simulink model "TRAS_PID_Pitch"  (R2016a)
settings: Solver=ode5  SolverMode=SingleTasking  StartTime=0.0  StopTime=90  FixedStep=0.01  RelTol=1e-3  AbsTol=1e-6
settings Model: SimulationMode=external  ExtModeTrigDuration=12000  ExtModeTrigLevel=0.400000  Creator=jims  LastModifiedBy=inteco
settings DataIOCC: ExternalInput=[]  InitialState=[]  MaxDataPoints=5000  SaveFormat=Array  SignalLoggingSaveFormat=ModelDataLogs  SaveOutput=off  SaveTime=off  SignalLoggingName=sigsOut
settings OptimizationCC: BooleanDataType=off  ExpressionDepthLimit=2147483647  InitFltsAndDblsToZero=on
settings DebuggingCC: SaveWithParameterizedLinksMsg=none  UnderspecifiedInitializationDetection=Classic  MergeDetectMultiDrivingBlocksExec=none  SignalResolutionControl=TryResolveAllWithWarning  MultiTaskDSMMsg=warning  MultiTaskCondExecSysMsg=none  IntegerOverflowMsg=none  FcnCallInpInsideContextMsg=UseLocalSettings  StateNameClashWarn=warning  IntegerSaturationMsg=none
settings HardwareCC: ProdBitPerPointer=32  ProdLargestAtomicFloat=None  ProdIntDivRoundTo=Undefined  ProdEndianess=Unspecified  ProdWordSize=32  ProdHWDeviceType=32-bit Generic
settings ModelReferenceCC: PropagateSignalLabelsOutOfModel=off
settings RTWCC: SystemTargetFile=rtcon_tras_usb2.tlc  TemplateMakefile=rtcon_tras_vc_usb2_x64.tmf  Description=TRAS RTDAC/USB2 (Visual C/C++)
settings STFCustomTargetCC: ModelReferenceCompliant=off  GeneratePreprocessorConditionals=Disable all  CombineOutputUpdateFcns=on  MatFileLogging=on  CPPClassGenCompliant=on  GRTInterface=off  SystemTargetFile=rtcon_tras_usb2.tlc
settings GRTTargetCC: ModelReferenceCompliant=off  ParMdlRefBuildCompliant=off  CompOptLevelCompliant=off  ConcurrentExecutionCompliant=off  UseToolchainInfoCompliant=off  ExtMode=on  ExtModeMexFile=rtcon_ext_comm
settings ConfigComp: CovModelRefEnable=Off  CovSFcnEnable=off

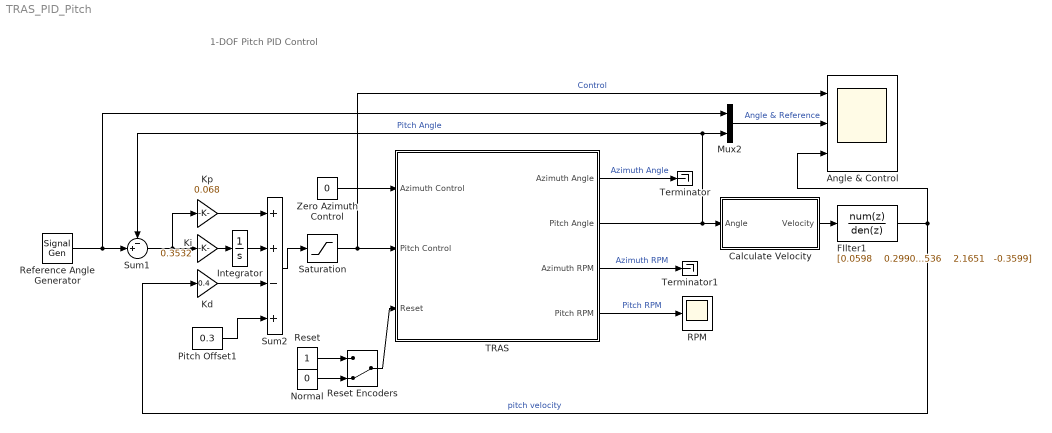
== system TRAS_PID_Pitch ==
  note: 1-DOF Pitch PID Control
  Angle & Control : Scope  NumInputPorts=3
  Calculate Velocity : Subsystem
      mask Display: disp( 'rad-to-rad/s' )
  FIlter1 : DiscreteTransferFcn  Numerator="[0.0598    0.2990    0.5980    0.5980    0.2990    0.0598] * 1e-3"  Denominator="[1.0000   -3.9845    6.4349   -5.2536    2.1651   -0.3599]"  SampleTime=0.01
  Integrator : Integrator  LimitOutput=on  UpperSaturationLimit=1.1  LowerSaturationLimit=-1.1
  Kd : Gain  Gain=0.4  SaturateOnIntegerOverflow=on  OutDataTypeStr=Inherit: Same as input  ParamDataTypeStr=Inherit: Same as input
  Ki : Gain  Gain=0.3532  SaturateOnIntegerOverflow=on  OutDataTypeStr=Inherit: Same as input  ParamDataTypeStr=Inherit: Same as input
  Kp : Gain  Gain=0.068  SaturateOnIntegerOverflow=on  OutDataTypeStr=Inherit: Same as input  ParamDataTypeStr=Inherit: Same as input
  Mux2 : Mux  Inputs=2
  Normal : Constant  Value=0
  Pitch Offset1 : Constant  Value=0.3
  RPM : Scope
  Reference Angle Generator : SignalGenerator  WaveForm=square  Amplitude=0.2  Frequency=1/50
  Reset : Constant
  Reset Encoders : ManualSwitch  CurrentSetting=0
  Saturation : Saturate  UpperLimit=1  LowerLimit=0
  Sum1 : Sum  Inputs=-+|  SaturateOnIntegerOverflow=on  InputSameDT=on  OutDataTypeStr=Inherit: Same as first input
  Sum2 : Sum  Inputs=++-+  SaturateOnIntegerOverflow=on  InputSameDT=on  OutDataTypeStr=Inherit: Same as first input
  TRAS : Subsystem
      mask Display: image(imread('Tras.JPG'))
  Terminator : Terminator
  Terminator1 : Terminator
  Zero Azimuth Control : Constant  Value=0
  wires:
  TRAS/1(Azimuth Angle) -> Terminator/1  "Azimuth Angle"
  TRAS/2(Pitch Angle) -> Sum1/1, Mux2/2, Calculate Velocity/1(Angle)  "Pitch Angle"
  TRAS/3(Azimuth RPM) -> Terminator1/1  "Azimuth RPM"
  TRAS/4(Pitch RPM) -> RPM/1  "Pitch RPM"
  Normal/1 -> Reset Encoders/2
  Reset/1 -> Reset Encoders/1
  Reset Encoders/1 -> TRAS/3(Reset)
  Sum1/1 -> Ki/1, Kp/1
  Reference Angle Generator/1 -> Mux2/1, Sum1/2
  Mux2/1 -> Angle & Control/2  "Angle & Reference"
  Zero Azimuth Control/1 -> TRAS/1(Azimuth Control)
  Saturation/1 -> Angle & Control/1, TRAS/2(Pitch Control)  "Control"
  Calculate Velocity/1(Velocity) -> FIlter1/1
  FIlter1/1 -> Angle & Control/3, Kd/1  "pitch velocity"
  Kp/1 -> Sum2/1
  Integrator/1 -> Sum2/2
  Ki/1 -> Integrator/1
  Sum2/1 -> Saturation/1
  Pitch Offset1/1 -> Sum2/4
  Kd/1 -> Sum2/3

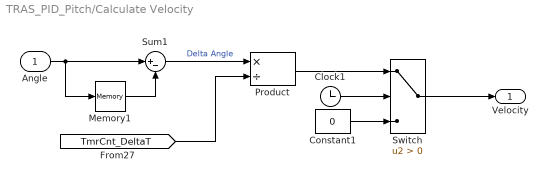
== system TRAS_PID_Pitch/Calculate Velocity ==
  Angle : Inport
  Clock1 : Clock
  Constant1 : Constant  Value=0
  Memory1 : Memory
  Product : Product  Inputs=*/  SaturateOnIntegerOverflow=on  InputSameDT=on  OutDataTypeStr=Inherit: Same as first input
  Sum1 : Sum  Inputs=|+-  SaturateOnIntegerOverflow=on  InputSameDT=on  OutDataTypeStr=Inherit: Same as first input
  Switch : Switch  Criteria=u2 > Threshold  SaturateOnIntegerOverflow=on  InputSameDT=on
  Velocity : Outport
  wires:
  [TmrCnt_DeltaT] -> Product/2
  Memory1/1 -> Sum1/2
  Angle/1 -> Sum1/1, Memory1/1
  Sum1/1 -> Product/1  "Delta Angle"
  Product/1 -> Switch/1
  Clock1/1 -> Switch/2
  Constant1/1 -> Switch/3
  Switch/1 -> Velocity/1

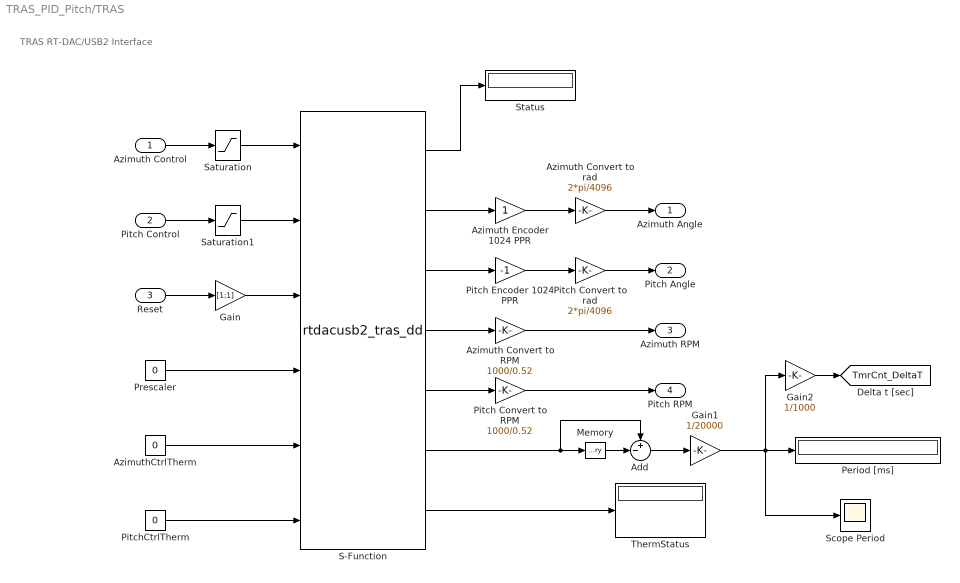
== system TRAS_PID_Pitch/TRAS ==
  note: TRAS RT-DAC/USB2
      | Interface
  Azimuth Control : Inport
  Pitch Control : Inport  Port=2
  Reset : Inport  Port=3
  Add : Sum  Inputs=+-|
  Azimuth Convert to RPM : Gain  Gain=1000/0.52  SaturateOnIntegerOverflow=on  OutDataTypeStr=Inherit: Same as input  ParamDataTypeStr=Inherit: Same as input
  Azimuth Convert to rad : Gain  Gain=2*pi/4096  SaturateOnIntegerOverflow=on  OutDataTypeStr=Inherit: Same as input  ParamDataTypeStr=Inherit: Same as input
  Azimuth Encoder 1024 PPR : Gain  SaturateOnIntegerOverflow=on  OutDataTypeStr=Inherit: Same as input  ParamDataTypeStr=Inherit: Same as input
  AzimuthCtrlTherm : Constant  Value=0
  Gain : Gain  Gain=[1;1]
  Gain1 : Gain  Gain=1/20000
  Gain2 : Gain  Gain=1/1000
  Memory : Memory
  Period [ms] : Display
  Pitch Convert to RPM : Gain  Gain=1000/0.52  SaturateOnIntegerOverflow=on  OutDataTypeStr=Inherit: Same as input  ParamDataTypeStr=Inherit: Same as input
  Pitch Convert to rad : Gain  Gain=2*pi/4096  SaturateOnIntegerOverflow=on  OutDataTypeStr=Inherit: Same as input  ParamDataTypeStr=Inherit: Same as input
  Pitch Encoder 1024 PPR : Gain  Gain=-1  SaturateOnIntegerOverflow=on  OutDataTypeStr=Inherit: Same as input  ParamDataTypeStr=Inherit: Same as input
  PitchCtrlTherm : Constant  Value=0
  Prescaler : Constant  Value=0
  S-Function : S-Function  FunctionName=rtdacusb2_tras_dd  Parameters=1, 0.01  SFunctionDeploymentMode=off  EnableBusSupport=off
  Saturation : Saturate  UpperLimit=1  LowerLimit=-1
  Saturation1 : Saturate  UpperLimit=1  LowerLimit=-1
  Scope Period : Scope
  Status : Display
  ThermStatus : Display
  Azimuth Angle : Outport
  Pitch Angle : Outport  Port=2
  Azimuth RPM : Outport  Port=3
  Pitch RPM : Outport  Port=4
  tag scope: TmrCnt_DeltaT=global
  wires:
  Gain2/1 -> [TmrCnt_DeltaT]
  Gain1/1 -> Gain2/1, Period [ms]/1, Scope Period/1
  S-Function/6 -> Add/1, Memory/1
  Add/1 -> Gain1/1
  Memory/1 -> Add/2
  S-Function/7 -> ThermStatus/1
  Pitch Convert to RPM/1 -> Pitch RPM/1
  Azimuth Convert to RPM/1 -> Azimuth RPM/1
  S-Function/5 -> Pitch Convert to RPM/1
  S-Function/4 -> Azimuth Convert to RPM/1
  Pitch Convert to rad/1 -> Pitch Angle/1
  S-Function/3 -> Pitch Encoder 1024 PPR/1
  Pitch Encoder 1024 PPR/1 -> Pitch Convert to rad/1
  Azimuth Convert to rad/1 -> Azimuth Angle/1
  S-Function/2 -> Azimuth Encoder 1024 PPR/1
  Azimuth Encoder 1024 PPR/1 -> Azimuth Convert to rad/1
  S-Function/1 -> Status/1
  Gain/1 -> S-Function/3
  Saturation1/1 -> S-Function/2
  Saturation/1 -> S-Function/1
  PitchCtrlTherm/1 -> S-Function/6
  AzimuthCtrlTherm/1 -> S-Function/5
  Prescaler/1 -> S-Function/4
  Reset/1 -> Gain/1
  Pitch Control/1 -> Saturation1/1
  Azimuth Control/1 -> Saturation/1
